simulink model "celect_controller"  (Simulink 7.1)
settings: Solver=ode45  StartTime=0.0  StopTime=150  RelTol=1e-3
settings Model: Creator=lv  LastModifiedBy=lv

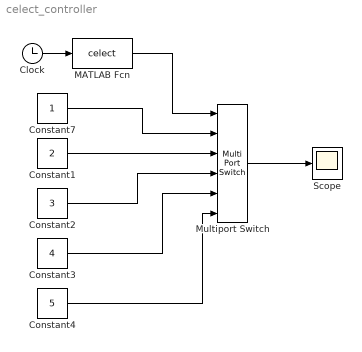
== system celect_controller ==
  Clock : Clock
      settings: Decimation=10
  Constant1 : Constant  Value=2  OutDataType=sfix(16)  OutScaling=2^0
  Constant2 : Constant  Value=3  OutDataType=sfix(16)  OutScaling=2^0
  Constant3 : Constant  Value=4  OutDataType=sfix(16)  OutScaling=2^0
  Constant4 : Constant  Value=5  OutDataType=sfix(16)  OutScaling=2^0
  Constant7 : Constant  OutDataType=sfix(16)  OutScaling=2^0
  MATLAB Fcn : MATLABFcn  MATLABFcn=celect
  Multiport Switch : MultiPortSwitch  Inputs=5  OutDataType=sfix(16)  OutScaling=2^0
  Scope : Scope
  wires:
  Multiport Switch/1 -> Scope/1
  Clock/1 -> MATLAB Fcn/1
  MATLAB Fcn/1 -> Multiport Switch/1
  Constant7/1 -> Multiport Switch/2
  Constant1/1 -> Multiport Switch/3
  Constant2/1 -> Multiport Switch/4
  Constant3/1 -> Multiport Switch/5
  Constant4/1 -> Multiport Switch/6
